simulink model "mo_phong_hsmc_2"  (R2025a)
settings: Solver=ode15s  StartTime=0.0  StopTime=60  RelTol=1e-3
model workspace: external: MATLAB File D:\EE4921E\new_hsmc\parameters.m (data not in the file)
undefined symbols (not defined in the file): para
settings Model: Creator=ADMIN88  LastModifiedBy=ADMIN88
settings DebuggingCC: UnderSpecifiedDimensionMsg=error

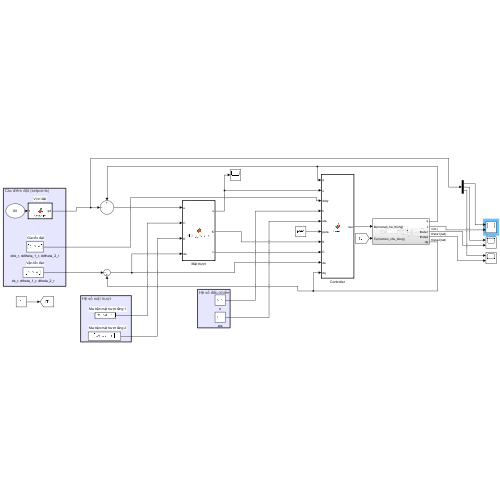
[thumbnail: Simulink's stored preview of the top-level diagram]
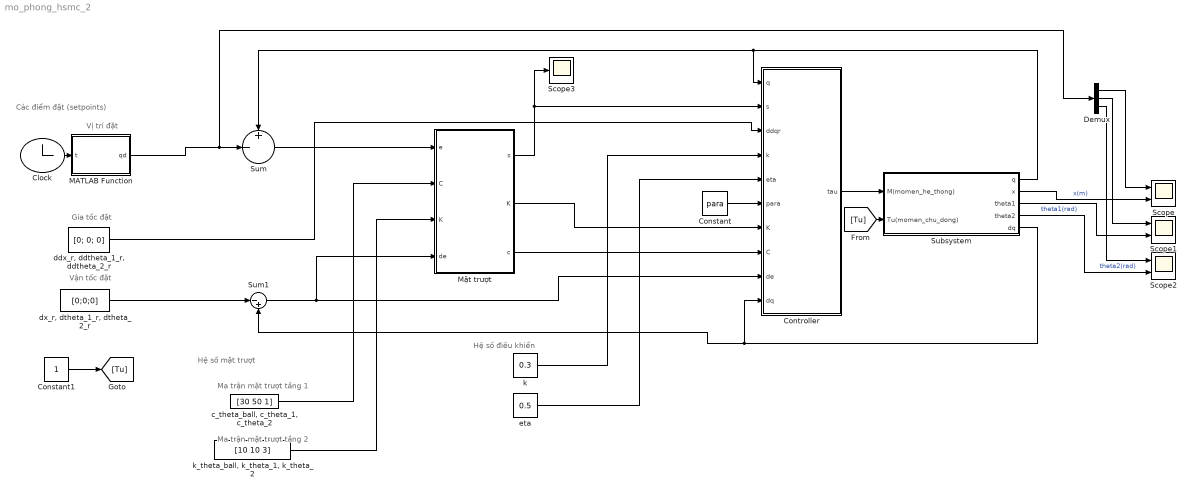
== system mo_phong_hsmc_2 ==
  note: Hệ số mặt trượt
  note: Ma trận mặt trượt tầng 2
  note: Gia tốc đặt
  note: Các điểm đặt (setpoints)
  note: Ma trận mặt trượt tầng 1
  note: Vị trí đặt
  note: Vận tốc đặt
  note: Hệ số điều khiển
  Clock : Clock
      settings: Decimation=2
  Constant : Constant  Value=para
  Constant1 : Constant
  Controller : MATLAB Function  TreatAsAtomicUnit=on
  Demux : Demux  Outputs=3
  MATLAB Function : MATLAB Function  TreatAsAtomicUnit=on
  Mặt trượt : MATLAB Function  TreatAsAtomicUnit=on
  Scope : Scope  NumInputPorts=2
      settings: ActiveDisplayYMinimum=-0.38203939447159713  ActiveDisplayYMaximum=2.478603730758385
  Scope1 : Scope  NumInputPorts=2
      settings: ActiveDisplayYMinimum=-0.019390477257063107  ActiveDisplayYMaximum=0.01781724568796134
  Scope2 : Scope  NumInputPorts=2
      settings: ActiveDisplayYMinimum=-1  ActiveDisplayYMaximum=1  DataLoggingVariableName=ScopeData2
  Scope3 : Scope
      settings: ActiveDisplayYMinimum=-4831.4458108419285  ActiveDisplayYMaximum=3483.0122975773584  DataLoggingVariableName=ScopeData3
  Subsystem : Subsystem
  Sum : Sum  Inputs=+|-||
  Sum1 : Sum  Inputs=|-+
  "c_theta_ball, c_theta_1, c_theta_2" : Constant  Value=[30 50 1]
  "ddx_r, ddtheta_1_r, ddtheta_2_r" : Constant  Value=[0; 0; 0]
  "dx_r, dtheta_1_r, dtheta_2_r" : Constant  Value=[0;0;0]
  eta : Constant  Value=0.5
  k : Constant  Value=0.3
  "k_theta_ball, k_theta_1, k_theta_2" : Constant  Value=[10 10 3]
  wires:
  Mặt trượt/1(s) -> Scope3/1, Controller/2(s)
  Controller/1(tau) -> Subsystem/1(M(momen_he_thong))
  Subsystem/1(q) -> Sum/1, Controller/1(q)
  Mặt trượt/3(c) -> Controller/8(C)
  Subsystem/5(dq) -> Sum1/2, Controller/10(dq)
  MATLAB Function/1(qd) -> Demux/1, Sum/2
  Sum/1 -> Mặt trượt/1(e)
  "c_theta_ball, c_theta_1, c_theta_2"/1 -> Mặt trượt/2(C)
  "k_theta_ball, k_theta_1, k_theta_2"/1 -> Mặt trượt/3("K ")
  Sum1/1 -> Controller/9(de), Mặt trượt/4(de)
  Mặt trượt/2(K) -> Controller/7(K)
  k/1 -> Controller/4(k)
  eta/1 -> Controller/5(eta)
  Constant/1 -> Controller/6(para)
  Subsystem/2(x) -> Scope/2  "x(m)"
  Subsystem/3(theta1) -> Scope1/2  "theta1(rad)"
  Subsystem/4(theta2) -> Scope2/2  "theta2(rad)"
  Clock/1 -> MATLAB Function/1(t)
  Demux/1 -> Scope/1
  Demux/2 -> Scope1/1
  Demux/3 -> Scope2/1
  Constant1/1 -> [Tu]
  [Tu] -> Subsystem/2(Tu(momen_chu_dong))
  "ddx_r, ddtheta_1_r, ddtheta_2_r"/1 -> Controller/3(ddqr)
  "dx_r, dtheta_1_r, dtheta_2_r"/1 -> Sum1/1

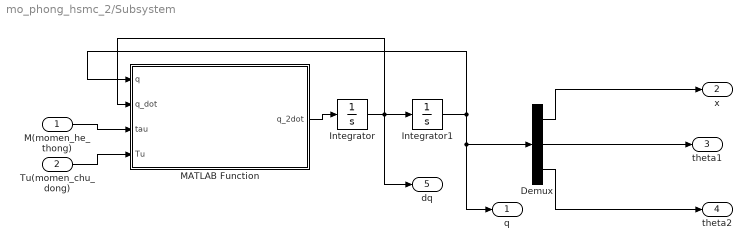
== system mo_phong_hsmc_2/Subsystem ==
  M(momen_he_thong) : Inport
  Tu(momen_chu_dong) : Inport  Port=2
  Demux : Demux  Outputs=3
  Integrator : Integrator  InitialCondition=[0;0;0]
  Integrator1 : Integrator  InitialCondition=[0;0.01;0]
  MATLAB Function : MATLAB Function  TreatAsAtomicUnit=on
  q : Outport
  x : Outport  Port=2
  theta1 : Outport  Port=3
  theta2 : Outport  Port=4
  dq : Outport  Port=5
  wires:
  Tu(momen_chu_dong)/1 -> MATLAB Function/4(Tu)
  Integrator1/1 -> MATLAB Function/1(q), q/1, Demux/1
  Demux/3 -> theta2/1
  Integrator/1 -> MATLAB Function/2(q_dot), dq/1, Integrator1/1
  M(momen_he_thong)/1 -> MATLAB Function/3(tau)
  Demux/1 -> x/1
  MATLAB Function/1(q_2dot) -> Integrator/1
  Demux/2 -> theta1/1

== matlab function mo_phong_hsmc_2/Controller ==
  data: q input; s input; tau output; ddqr input; k input; eta input; para input; K input size=[1 3]; C input size=[3 3]; de input size=[3 1]; dq input
function tau  = hsmc(q,s, ddqr, k, eta, para,K,C,de, dq)
%% Thông số mô hình
mb = para(1); 
mt1 = para(2);
mt2 = para(3);
Jb = para(4);
Jx = para(5);
Jt1 = para(6);
Jt2 = para(7);
rb = para(8);
rx = para(9);
l1 = para(10);
l2 = para(11);
h = para(12);
g = para(13);
ks = para(14);
bs = para(15);

%% Biến trạng thái
x = q(1);
th1 = q(2);
th2 = q(3);
dx = dq(1);
dth1 = dq(2);
dth2 = dq(3);

%% Các ma trận mô hình
m11=mb+mt1+mt2+Jb/(rb^2)+Jx/(rx^2);
m22=Jt1+Jt2+Jx+h^2*mt2+l1^2*mt1+l2^2*mt2+(2*Jx*rx)/rb+Jx*(rb^2)/(rx^2)+2*h*l2*mt2*cos(th2);
m33=mt2*l2^2+Jt2;
m12=h*mt2*cos(th1)-(Jx*rb)/rx-Jx/rx+l1*mt1*cos(th1)+l2*mt2*cos(th1+th2);
m21=m12;
m13=l2*mt2*cos(th1+th2);
m31=m13;
m23=mt2*l2^2+h*mt2*l2*cos(th2)+Jt2;
m32=m23;
M=[m11 m12 m13; m21 m22 m23; m31 m32 m33];

n11=-mt2*(2*h*dth1^2*sin(th1)+2*l2*(dth1+dth2)^2*sin(th1+th2))/2-l1*mt1*dth1^2*sin(th1);
n21=-h*l2*mt2*dth2^2*sin(th2)-2*h*l2*mt2*dth2*dth1*sin(th2)-g*l2*mt2*sin(th1+th2)-g*h*mt2*sin(th1)-g*l1*mt1*sin(th1);
n31=h*l2*mt2*dth1^2*sin(th2)+ks*th2-g*l2*mt2*sin(th1+th2);
N=[n11; n21; n31];

j11=1/rx;
j21=-(1+rb/rx);
j31=0;
J=[j11; j21; j31];

%Q_active=[0; bs*dth2 ; bs*dth2];
%% Các hàm của model
%f = -M^(-1)*Q_active-M^(-1)*N;
f= -M^(-1)*N;
g = M^(-1)*J;

%% Các hàm phụ trợ
al=K*(f-ddqr+C*de);
be=K*g;

%% Disturbace guess:
Tu_min=-2;
Tu_max=2;
Tu_1=(Tu_max-Tu_min)/2;
Tu_2=(Tu_max+Tu_min)/2;
Tu_c=Tu_2-Tu_1*sign(s);
%% Control signal
tau=1/be*(-k*s-eta*sign(s)-al-K*M^(-1)*Tu_c*[0; 1; 1]);
%tau=1/be*(-k*s-eta*sign(s)-al);

== matlab function mo_phong_hsmc_2/Subsystem/MATLAB Function ==
  data: q input; q_dot input; tau input; q_2dot output size=[3 1]; Tu input
function  q_2dot= Ballbot2D(q, q_dot, tau, Tu)
mb = 0.62; 
mt1 = 40;
mt2 = 35;
Jb = 6.5*10e-3;
Jx = 0.15*10e-3;
Jt1 = 1.6;
Jt2 = 1.18;
rb = 0.125;
rx = 0.05;
l1 = 0.57;
l2 = 0.32;
h = 0.6;
g = 9.81;
ks = 850;
bs = 350;

x = q(1);
th1 = q(2);
th2 = q(3);
dx = q_dot(1);
dth1 = q_dot(2);
dth2 = q_dot(3);

m11=mb+mt1+mt2+Jb/(rb^2)+Jx/(rx^2);
m22=Jt1+Jt2+Jx+h^2*mt2+l1^2*mt1+l2^2*mt2+(2*Jx*rx)/rb+Jx*(rb^2)/(rx^2)+2*h*l2*mt2*cos(th2);
m33=mt2*l2^2+Jt2;
m12=h*mt2*cos(th1)-(Jx*rb)/rx-Jx/rx+l1*mt1*cos(th1)+l2*mt2*cos(th1+th2);
m21=m12;
m13=l2*mt2*cos(th1+th2);
m31=m13;
m23=mt2*l2^2+h*mt2*l2*cos(th2)+Jt2;
m32=m23;
M=[m11 m12 m13; m21 m22 m23; m31 m32 m33];

n11=-mt2*(2*h*dth1^2*sin(th1)+2*l2*(dth1+dth2)^2*sin(th1+th2))/2-l1*mt1*dth1^2*sin(th1);
n21=-h*l2*mt2*dth2^2*sin(th2)-2*h*l2*mt2*dth2*dth1*sin(th2)-g*l2*mt2*sin(th1+th2)-g*h*mt2*sin(th1)-g*l1*mt1*sin(th1);
n31=h*l2*mt2*dth1^2*sin(th2)+ks*th2-g*l2*mt2*sin(th1+th2);
N=[n11; n21; n31];

j11=1/rx;
j21=-(1+rb/rx);
j31=0;
J=[j11; j21; j31];

q11=0;
q21=Tu-bs*dth2;
q31=Tu-bs*dth2;
Q=[q11; q21; q31];

q_2dot=inv(M)*(J*tau+Q-N);
end

== matlab function mo_phong_hsmc_2/Mặt trượt ==
  data: e input size=[3 1]; C input size=[1 3]; K input size=[1 3]; s output; K output; de input size=[3 1]; c output
function [s, K, c] = sliding_surface(e, C, K, de)
c=diag(C);
s1=de+c*e;
s=K*s1;

== matlab function mo_phong_hsmc_2/MATLAB Function ==
  data: t input; qd output
function qd = setpoint(t)

%qd = [2*trapmf(t,[0;10;30;40]); 0; 0];
%qd = [2;0;0];
qd = [1+1*sin(0.25*t-pi/2); 0; 0];
